simulink subsystem "Day4_5_Scenario_1"  (R2024a)
settings: Solver=VariableStepAuto  StartTime=0.0  StopTime=10.0  RelTol=1e-3
libraries: CarMaker4SL x10
settings Model: Creator=junhyung.cha  LastModifiedBy=junhyung.cha

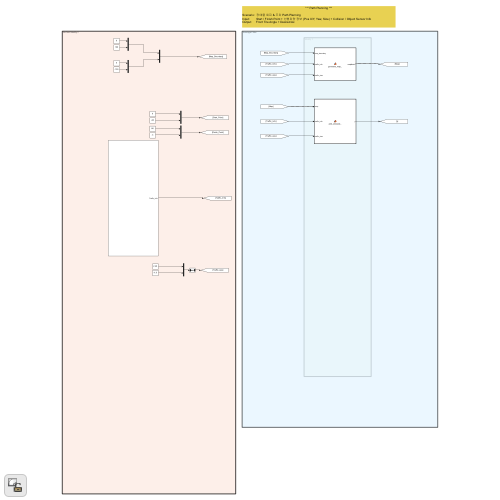
[thumbnail: Simulink's stored preview of the top-level diagram]
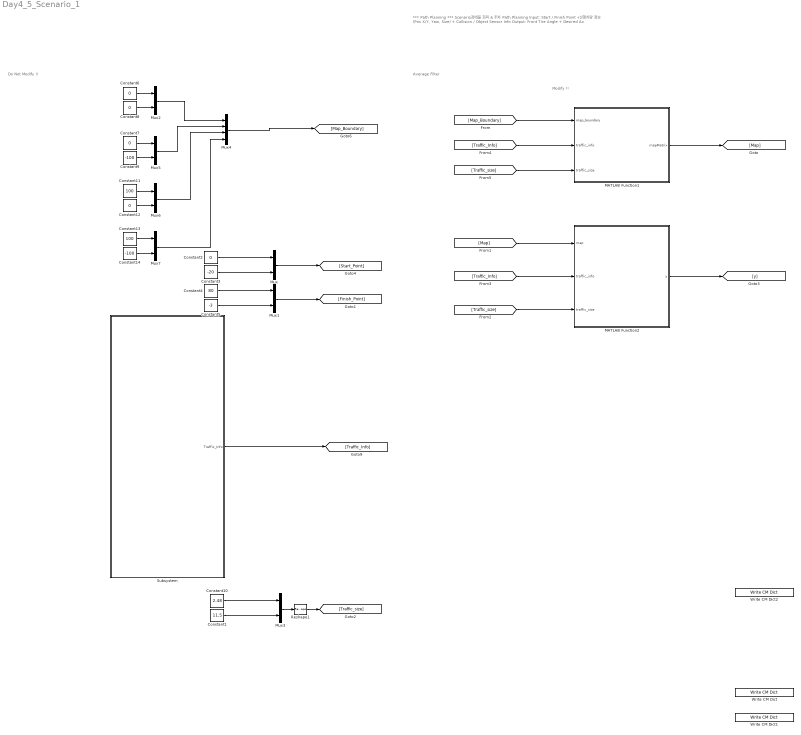
== system Day4_5_Scenario_1 ==
  note: Average Filter
  note: Do Not Modify !!
  note: Modify !!
  note: *** Path Planning ***
      |
      | Scenario: 장애물 회피 & 주차 Path Planning
      | Input: Start / Finish Point + 선행차량 정보 (Pos X/Y, Yaw, Size) + Collision / Object Sensor Info
      | Output: Front Tire Angle + Desired Ax
  Constant1 : Constant  Value=11.5
  Constant10 : Constant  Value=2.48
  Constant11 : Constant  Value=100
  Constant{2,6..8,12} (5 alike) : Constant  Value=0
  Constant13 : Constant  Value=100
  Constant14 : Constant  Value=-100
  Constant3 : Constant  Value=-20
  Constant4 : Constant  Value=80
  Constant5 : Constant  Value=-3
  Constant9 : Constant  Value=-100
  MATLAB Function1 : MATLAB Function  TreatAsAtomicUnit=on
  MATLAB Function2 : MATLAB Function  TreatAsAtomicUnit=on
  Mux{,1..3,5..7} (7 alike) : Mux  Inputs=2
  Mux4 : Mux
  Reshape1 : Reshape  OutputDimensionality=Row vector (2-D)  OutputDimensions=[2,2]
  Subsystem : Subsystem
  Write CM Dict : CarMaker4SL/Write CM Dict  xname=Car.CFL.rz_ext  xsync=off
  Write CM Dict1 : CarMaker4SL/Write CM Dict  xname=Car.CFR.rz_ext  xsync=off
  Write CM Dict2 : CarMaker4SL/Write CM Dict  xname=AccelCtrl.DesiredAx  xsync=off
  wires:
  [Map] -> MATLAB Function2/1(map)
  Mux/1 -> [Start_Point]
  Constant2/1 -> Mux/1
  Constant3/1 -> Mux/2
  Constant5/1 -> Mux1/2
  Mux1/1 -> [Finish_Point]
  Constant4/1 -> Mux1/1
  Constant6/1 -> Mux2/1
  Constant8/1 -> Mux2/2
  Constant9/1 -> Mux5/2
  [Map_Boundary] -> MATLAB Function1/1(map_boundary)
  Subsystem/1(Traffic_Info) -> [Traffic_Info]
  [Traffic_Info] -> MATLAB Function2/2(traffic_info)
  Mux3/1 -> Reshape1/1
  [Traffic_size] -> MATLAB Function2/3(traffic_size)
  Constant10/1 -> Mux3/1
  Constant1/1 -> Mux3/2
  Mux2/1 -> Mux4/1
  Mux5/1 -> Mux4/2
  Mux4/1 -> [Map_Boundary]
  Constant7/1 -> Mux5/1
  [Traffic_Info] -> MATLAB Function1/2(traffic_info)
  [Traffic_size] -> MATLAB Function1/3(traffic_size)
  Reshape1/1 -> [Traffic_size]
  MATLAB Function1/1(mapMatrix) -> [Map]
  MATLAB Function2/1(y) -> [y]
  Constant11/1 -> Mux6/1
  Mux6/1 -> Mux4/3
  Constant12/1 -> Mux6/2
  Constant14/1 -> Mux7/2
  Mux7/1 -> Mux4/4
  Constant13/1 -> Mux7/1

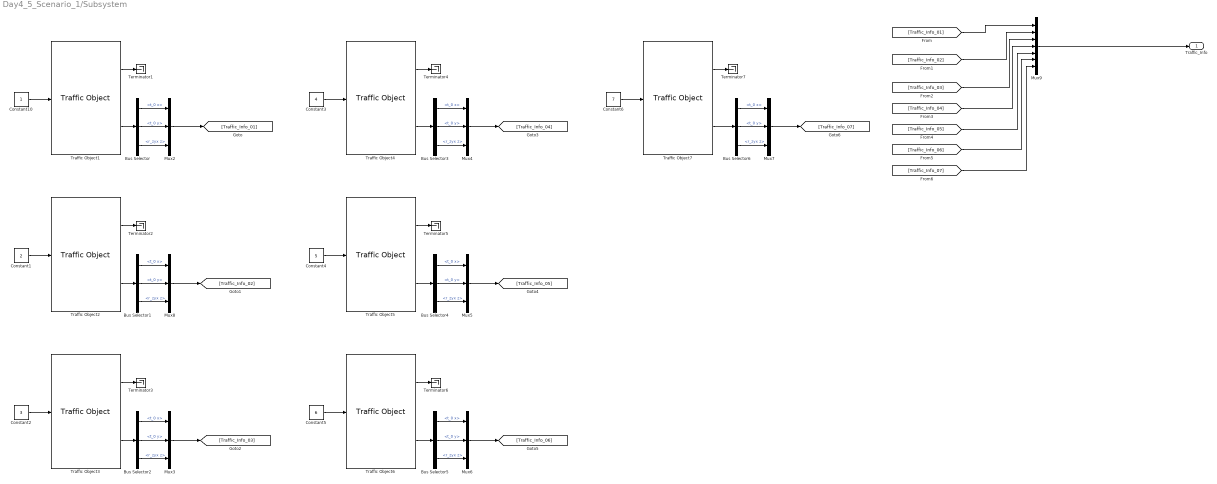
== system Day4_5_Scenario_1/Subsystem ==
  Bus Selector{,1..6} (7 alike) : BusSelector  OutputSignals=t_0 x,t_0 y,r_zyx z
  Constant1 : Constant  Value=2
  Constant10 : Constant
  Constant2 : Constant  Value=3
  Constant3 : Constant  Value=4
  Constant4 : Constant  Value=5
  Constant5 : Constant  Value=6
  Constant6 : Constant  Value=7
  Mux{2..8} (7 alike) : Mux  Inputs=3
  Mux9 : Mux  Inputs=7
  Terminator{1..7} (7 alike) : Terminator
  Traffic Object1 : CarMaker4SL/Traffic Object  xname=T01  ximode=Traffic Id  xstime=Inherited
      settings: SourceProductName=CarMaker4SL
  Traffic Object2 : CarMaker4SL/Traffic Object  xname=T02  ximode=Traffic Id  xstime=Inherited
      settings: SourceProductName=CarMaker4SL
  Traffic Object3 : CarMaker4SL/Traffic Object  xname=T03  ximode=Traffic Id  xstime=Inherited
      settings: SourceProductName=CarMaker4SL
  Traffic Object4 : CarMaker4SL/Traffic Object  xname=T04  ximode=Traffic Id  xstime=Inherited
      settings: SourceProductName=CarMaker4SL
  Traffic Object5 : CarMaker4SL/Traffic Object  xname=T05  ximode=Traffic Id  xstime=Inherited
      settings: SourceProductName=CarMaker4SL
  Traffic Object6 : CarMaker4SL/Traffic Object  xname=T06  ximode=Traffic Id  xstime=Inherited
      settings: SourceProductName=CarMaker4SL
  Traffic Object7 : CarMaker4SL/Traffic Object  xname=T07  ximode=Traffic Id  xstime=Inherited
      settings: SourceProductName=CarMaker4SL
  Traffic_Info : Outport
  wires:
  [Traffic_Info_07] -> Mux9/7
  [Traffic_Info_06] -> Mux9/6
  [Traffic_Info_05] -> Mux9/5
  [Traffic_Info_04] -> Mux9/4
  [Traffic_Info_03] -> Mux9/3
  Mux9/1 -> Traffic_Info/1
  [Traffic_Info_02] -> Mux9/2
  [Traffic_Info_01] -> Mux9/1
  Mux2/1 -> [Traffic_Info_01]
  Traffic Object7/2 -> Bus Selector6/1
  Bus Selector6/3 -> Mux7/3  "<r_zyx z>"
  Bus Selector6/1 -> Mux7/1  "<t_0 x>"
  Mux7/1 -> [Traffic_Info_07]
  Bus Selector6/2 -> Mux7/2  "<t_0 y>"
  Traffic Object6/2 -> Bus Selector5/1
  Bus Selector5/3 -> Mux6/3  "<r_zyx z>"
  Bus Selector5/1 -> Mux6/1  "<t_0 x>"
  Mux6/1 -> [Traffic_Info_06]
  Bus Selector5/2 -> Mux6/2  "<t_0 y>"
  Traffic Object5/2 -> Bus Selector4/1
  Bus Selector4/3 -> Mux5/3  "<r_zyx z>"
  Bus Selector4/1 -> Mux5/1  "<t_0 x>"
  Mux5/1 -> [Traffic_Info_05]
  Bus Selector4/2 -> Mux5/2  "<t_0 y>"
  Traffic Object4/2 -> Bus Selector3/1
  Bus Selector3/3 -> Mux4/3  "<r_zyx z>"
  Bus Selector3/1 -> Mux4/1  "<t_0 x>"
  Mux4/1 -> [Traffic_Info_04]
  Bus Selector3/2 -> Mux4/2  "<t_0 y>"
  Traffic Object3/2 -> Bus Selector2/1
  Bus Selector2/3 -> Mux3/3  "<r_zyx z>"
  Bus Selector2/1 -> Mux3/1  "<t_0 x>"
  Mux3/1 -> [Traffic_Info_03]
  Bus Selector2/2 -> Mux3/2  "<t_0 y>"
  Traffic Object2/2 -> Bus Selector1/1
  Bus Selector1/3 -> Mux8/3  "<r_zyx z>"
  Bus Selector1/1 -> Mux8/1  "<t_0 x>"
  Mux8/1 -> [Traffic_Info_02]
  Bus Selector1/2 -> Mux8/2  "<t_0 y>"
  Bus Selector/3 -> Mux2/3  "<r_zyx z>"
  Bus Selector/2 -> Mux2/2  "<t_0 y>"
  Bus Selector/1 -> Mux2/1  "<t_0 x>"
  Traffic Object1/2 -> Bus Selector/1
  Traffic Object7/1 -> Terminator7/1
  Constant6/1 -> Traffic Object7/1
  Constant5/1 -> Traffic Object6/1
  Traffic Object6/1 -> Terminator6/1
  Traffic Object5/1 -> Terminator5/1
  Constant4/1 -> Traffic Object5/1
  Constant3/1 -> Traffic Object4/1
  Traffic Object4/1 -> Terminator4/1
  Traffic Object3/1 -> Terminator3/1
  Constant2/1 -> Traffic Object3/1
  Constant1/1 -> Traffic Object2/1
  Traffic Object2/1 -> Terminator2/1
  Traffic Object1/1 -> Terminator1/1
  Constant10/1 -> Traffic Object1/1

== matlab function Day4_5_Scenario_1/MATLAB Function1 ==
  settings: sampleTime=0.05
  data: map_boundary input; mapMatrix output size=[1000, 1000]; traffic_info input; traffic_size input
function mapMatrix = generate_map_(map_boundary, traffic_info, traffic_size)
    mapMatrix = 0;
end

== matlab function Day4_5_Scenario_1/MATLAB Function2 ==
  settings: sampleTime=0.1
  data: map input; y output; traffic_info input; traffic_size input
function y = add_obstacle_(map, traffic_info, traffic_size)
    y = 0;
end
